simulink model "inverted_pendulum_PID_controller"  (R2022b)
settings: Solver=FixedStepAuto  StartTime=0.0  StopTime=10  FixedStep=0.001  RelTol=1e-3
undefined symbols (not defined in the file): F, g, Kd, L, m, M, thetastart, xstart
libraries: slpidlib x1
settings Model: Creator=Alex  LastModifiedBy=anton

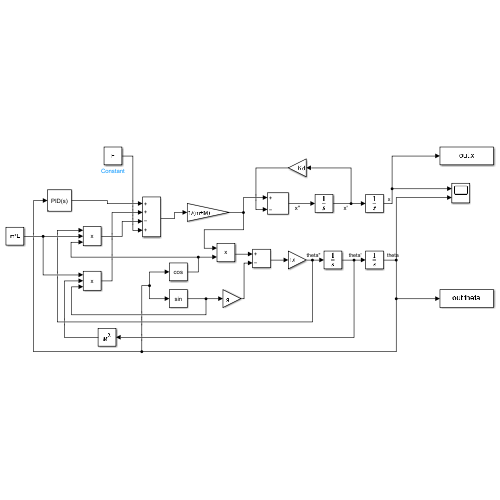
[thumbnail: Simulink's stored preview of the top-level diagram]
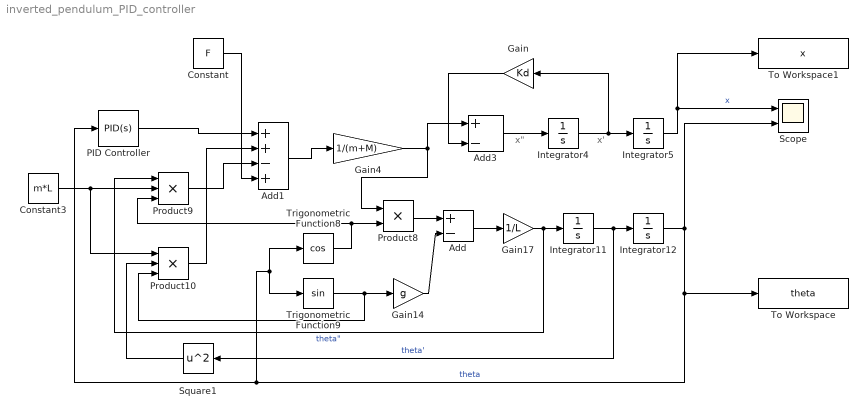
== system inverted_pendulum_PID_controller ==
  note: x'
  note: x"
  Add : Sum  Inputs=+-
  Add1 : Sum  Inputs=++-+
  Add3 : Sum  Inputs=+-
  Constant : Constant  Value=F
  Constant3 : Constant  Value=m*L
  Gain : Gain  Gain=Kd
  Gain14 : Gain  Gain=g
  Gain17 : Gain  Gain=1/L
  Gain4 : Gain  Gain=1/(m+M)
  Integrator11 : Integrator
  Integrator12 : Integrator  InitialCondition=thetastart
  Integrator4 : Integrator
  Integrator5 : Integrator  InitialCondition=xstart
  PID Controller : slpidlib/PID Controller  Controller=PID  Form=Parallel  TimeDomain=Continuous-time  UseExternalTs=off  SampleTime=-1  IntegratorMethod=Forward Euler  FilterMethod=Forward Euler  ControllerParametersSource=internal  P=-196  I=-110  UseKiTs=off  D=-75  N=292.386539928776  UseFilter=on  TunerSelectOption=Transfer Function Based (PID Tuner App)  InitialConditionSource=internal  InitialConditionForIntegrator=0  InitialConditionForFilter=0  DifferentiatorICPrevScaledInput=0  ExternalReset=none  TrackingMode=off  Kt=1  LimitOutput=off  SatLimitsSource=internal  UpperSaturationLimit=inf  LowerSaturationLimit=-inf  LinearizeAsGain=on  AntiWindupMode=none  Kb=1  LimitIntegrator=off  UpperIntegratorSaturationLimit=inf  LowerIntegratorSaturationLimit=-inf  POutMin=[]  POutMax=[]  IOutMin=[]  IOutMax=[]  DOutMin=[]  DOutMax=[]  NOutMin=[]  NOutMax=[]  SumOutMin=[]  SumOutMax=[]  SaturationOutMin=[]  SaturationOutMax=[]  PParamMin=[]  PParamMax=[]  IParamMin=[]  IParamMax=[]  DParamMin=[]  DParamMax=[]  NParamMin=[]  NParamMax=[]  KbParamMin=[]  KbParamMax=[]  KtParamMin=[]  KtParamMax=[]  KbOutMin=[]  KbOutMax=[]  KtOutMin=[]  KtOutMax=[]  IntegratorOutMin=[]  IntegratorOutMax=[]  FilterOutMin=[]  FilterOutMax=[]  SumI1OutMin=[]  SumI1OutMax=[]  SumI2OutMin=[]  SumI2OutMax=[]  SumI3OutMin=[]  SumI3OutMax=[]  SumI4OutMin=[]  SumI4OutMax=[]  SumDOutMin=[]  SumDOutMax=[]  DifferentiatorOutMin=[]  DifferentiatorOutMax=[]  FilterDiffOutCoefMin=[]  FilterDiffOutCoefMax=[]  ReciprocalOutMin=[]  ReciprocalOutMax=[]  SumDenOutMin=[]  SumDenOutMax=[]  SumNumOutMin=[]  SumNumOutMax=[]  DivideOutMin=[]  DivideOutMax=[]  UdiffTsProdOutMin=[]  UdiffTsProdOutMax=[]  NTsProdOutMin=[]  NTsProdOutMax=[]  UintegralTsProdOutMin=[]  UintegralTsProdOutMax=[]  UngainTsProdOutMin=[]  UngainTsProdOutMax=[]  ClampingZeroOutDataTypeStr=Inherit: Inherit via back propagation  ClampingZeroOutMin=[]  ClampingZeroOutMax=[]  FilterDenConstantOutDataTypeStr=Inherit: Inherit via back propagation  FilterDenConstantOutMin=[]  FilterDenConstantOutMax=[]  PCopyOutDataTypeStr=Inherit: Inherit via back propagation  PCopyOutMin=[]  PCopyOutMax=[]  NCopyOutDataTypeStr=Inherit: Inherit via back propagation  NCopyOutMin=[]  NCopyOutMax=[]  IntegratorContinuousStateAttributes=''  IntegratorStateMustResolveToSignalObject=off  IntegratorRTWStateStorageClass=Auto  FilterContinuousStateAttributes=''  FilterStateMustResolveToSignalObject=off  FilterRTWStateStorageClass=Auto  ParallelPVariant=InternalParameters  IdealPVariant=Disabled  IVariant=InternalParameters  DVariant=InternalParameters  IntegratorVariant=Continuous  SatVariant=Disabled  AWVariant=Passthrough  PCopyVariant=Disabled  TRVariant=Disabled  FdbkBlocksVariant=Forward  IdealPFdbkVariant=Disabled  SatFdbkVariant=Disabled  DerivativeFilterVariant=ContFilter  NVariant=InternalParameters  NCopyVariant=Disabled  FilterICVariant=InternalICsFilter  IntegratorICVariant=InternalICs  ExternalResetVariant=Disabled  TRSumVariant=Passthrough  SumFdbkVariant=Disabled  SumVariant=Sum_PID  TsampFilterVariant=InternalTs  TsampNgainVariant=Passthrough  TsampIntegralVariant=Passthrough  ExternalSaturationOutDataTypeStr=Inherit: Same as second input
  Product10 : Product  Inputs=3
  Product8 : Product
  Product9 : Product  Inputs=3
  Scope : Scope  NumInputPorts=2
  Square1 : Math  Operator=square
  To Workspace : ToWorkspace  VariableName=theta  SaveFormat=Timeseries  SampleTime=-1
  To Workspace1 : ToWorkspace  VariableName=x  SaveFormat=Timeseries  SampleTime=-1
  Trigonometric Function8 : Trigonometry  Operator=cos
  Trigonometric Function9 : Trigonometry
  wires:
  Add1/1 -> Gain4/1
  Constant3/1 -> Product9/2, Product10/1
  Square1/1 -> Product10/2
  Product8/1 -> Add/1
  Gain14/1 -> Add/2
  Integrator4/1 -> Gain/1, Integrator5/1
  Trigonometric Function9/1 -> Product10/3, Gain14/1
  Integrator5/1 -> To Workspace1/1, Scope/1  "x"
  Gain4/1 -> Add3/1, Product8/1
  Integrator11/1 -> Square1/1, Integrator12/1  "theta'"
  Gain17/1 -> Product9/1, Integrator11/1  "theta\""
  Add/1 -> Gain17/1
  Trigonometric Function8/1 -> Product9/3, Product8/2
  PID Controller/1 -> Add1/1
  Integrator12/1 -> To Workspace/1, PID Controller/1, Trigonometric Function9/1, Trigonometric Function8/1, Scope/2  "theta"
  Add3/1 -> Integrator4/1
  Gain/1 -> Add3/2
  Product9/1 -> Add1/3
  Product10/1 -> Add1/2
  Constant/1 -> Add1/4
